simulink model "Model_6DOF_B3"  (R2020b)
settings: Solver=FixedStepAuto  StartTime=0.0  StopTime=120  FixedStep=0.05  RelTol=1e-3
values from neighbouring files (symbols this model uses):
  Ba_0 = [0 0 0 0 0 0]    [ctrl_mode_param.m]
  Bb = 4418825.3321    [load_data.m]
  Bv_0 = [tgt_speed 0 0 0 0 0]    [ctrl_mode_param.m]
  Bx_0 = [0 0 tgt_depth 0 0 0]    [ctrl_mode_param.m]
  Ixx = 5.23e7    (= 52300000)    [load_data.m]
  Ixy = 0    [load_data.m]
  Ixz = 0    [load_data.m]
  Iyy = 1.375e9    (= 1375000000)    [load_data.m]
  Iyz = 0    [load_data.m]
  Izz = 1.367e9    (= 1367000000)    [load_data.m]
  Mb = 4418825.3321    [load_data.m]
  Xb = 0    [load_data.m]
  Xg = 0    [load_data.m]
  Yb = 0    [load_data.m]
  Yg = 0    [load_data.m]
  Zb = 0.4406    [load_data.m]
  Zg = 0    [load_data.m]
undefined symbols (not defined in the file or in its folder): dA_BP1, dA_BP2, dA_Hull, dA_PH, dA_Sail, dA_SProot, dA_X1a, dA_X1b, dA_X2a, dA_X2b, dA_X3a, dA_X3b, dA_X4a, dA_X4b, its, n_BP1, n_BP2, n_Hull, n_PH, n_Sail, n_SProot, n_X1a, n_X1b, n_X2a, n_X2b, n_X3a, n_X3b, n_X4a, n_X4b, nt_BP1, nt_BP2, nt_Hull, nt_PH, nt_Sail, nt_SProot, nt_X1a, nt_X1b, nt_X2a, nt_X2b, nt_X3a, nt_X3b, nt_X4a, nt_X4b, Usp, vt1_BP1, vt1_BP2, vt1_Hull, vt1_PH, vt1_Sail, vt1_SProot, vt1_X1a, vt1_X1b, vt1_X2a, vt1_X2b, vt1_X3a, vt1_X3b, vt1_X4a, vt1_X4b, vt2_BP1, vt2_BP2 ... (+27)
libraries: simulink x5
(part 4 of 15)

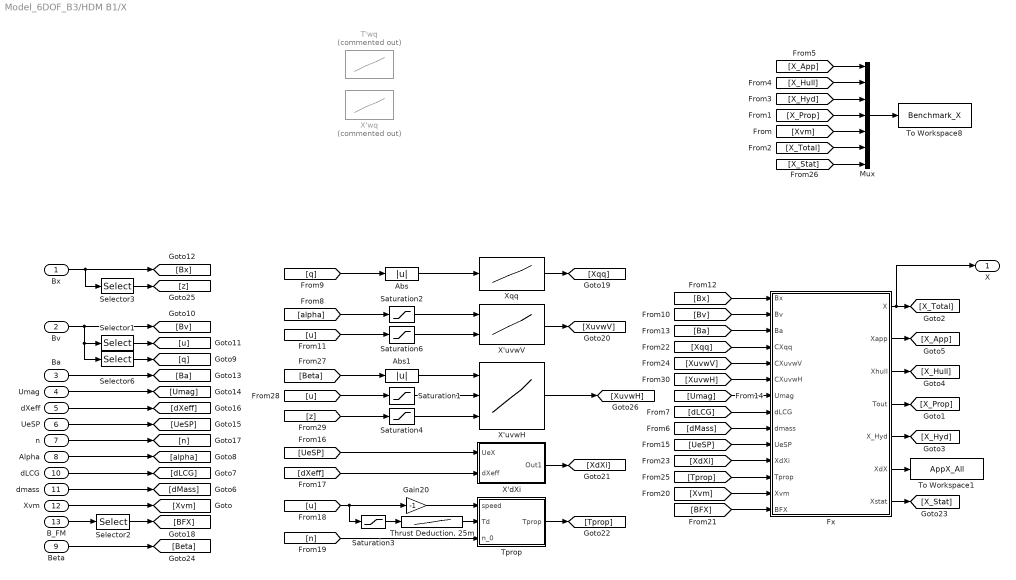
== system Model_6DOF_B3/HDM B1/X ==
  Bx : Inport
  Bv : Inport  Port=2
  Ba : Inport  Port=3
  Umag : Inport  Port=4
  dXeff : Inport  Port=5
  UeSP : Inport  Port=6
  n : Inport  Port=7
  Alpha : Inport  Port=8
  Beta : Inport  Port=9
  dLCG : Inport  Port=10
  dmass : Inport  Port=11
  Xvm : Inport  Port=12
  B_FM : Inport  Port=13
  Abs : Abs
  Abs1 : Abs
  Fx : MATLAB Function  TreatAsAtomicUnit=on
  Gain20 : Gain  Gain=-1
  Mux : Mux  Inputs=7
  Saturation1 : Saturate  UpperLimit=-1.543332  LowerLimit=-5.14444
  Saturation2 : Saturate  UpperLimit=30  LowerLimit=-30
  Saturation3 : Saturate  UpperLimit=-1.54333333  LowerLimit=-5.1444
  Saturation4 : Saturate  UpperLimit=-13.8724  LowerLimit=-35.0624
  Saturation6 : Saturate  UpperLimit=-1.543332  LowerLimit=-5.14444
  Selector1 : Selector  InputPortWidth=6  IndexOptions=Index vector (dialog)  Indices=1  OutputSizes=1
  Selector2 : Selector  InputPortWidth=6  IndexOptions=Index vector (dialog)  Indices=1  OutputSizes=1
  Selector3 : Selector  InputPortWidth=6  IndexOptions=Index vector (dialog)  Indices=3  OutputSizes=1
  Selector6 : Selector  InputPortWidth=6  IndexOptions=Index vector (dialog)  Indices=5  OutputSizes=1
  T'wq : Lookup_n-D  Commented=on  BreakpointsForDimension1=|  BreakpointsForDimension2=|  Table=|  InternalRulePriority=Speed  RndMeth=Simplest  InputSameDT=on
      BreakpointsForDimension1=|
      | [-2.5000E-02
      | -2.0000E-02
      | -1.5000E-02
      | -1.0000E-02
      | -5.0000E-03
      | 0.0000E+00
      | 5.0000E-03
      | ]
      BreakpointsForDimension2=|
      | [-7.71666
      | -5.14444
      | -3.086664]
      Table=|
      | reshape([-2.7354E-04
      | -2.2597E-04
      | -1.7840E-04
      | -1.3083E-04
      | -8.3252E-05
      | -3.5680E-05
      | 1.1893E-05
      | -9.4081E-05
      | -7.5784E-05
      | -5.7487E-05
      | -3.9189E-05
      | -2.0892E-05
      | -2.5949E-06
      | 1.5702E-05
      | -1.4962E-04
      | -1.2035E-04
      | -9.1070E-05
      | -6.1795E-05
      | -3.2519E-05
      | -3.2436E-06
      | 2.6032E-05
      | ],[7,3])
      settings: InputPortMap=u0,u1
  "Thrust Deduction, 25m" : Lookup_n-D  NumberOfTableDimensions=1  BreakpointsForDimension1=[-5.14444,-3.086664,-1.543332]  BreakpointsForDimension2=[0.1 1.543332 3.086664 5.14444 100]  Table=[0.2496,0.2444134,0.245958]  InternalRulePriority=Speed  RndMeth=Simplest  InputSameDT=on
  To Workspace1 : ToWorkspace  VariableName=AppX_All  SaveFormat=Timeseries  SampleTime=-1
  To Workspace8 : ToWorkspace  VariableName=Benchmark_X  SaveFormat=Timeseries  SampleTime=-1
  Tprop : MATLAB Function  TreatAsAtomicUnit=on
  X'dXi : Subsystem
  X'uvwH : Lookup_n-D  NumberOfTableDimensions=3  BreakpointsForDimension1=|  BreakpointsForDimension2=|  BreakpointsForDimension3=|  Table=|  InternalRulePriority=Speed  RndMeth=Simplest  InputSameDT=on
      BreakpointsForDimension1=|
      | [0
      | 4
      | 8
      | 12]
      BreakpointsForDimension2=|
      | [-5.1444
      | -3.08664
      | -1.54332]
      Table=|
      | reshape([0.0000000E+00
      | 8.7490400E-05
      | -4.2970032E-04
      | -8.6882993E-04
      | 0.0000000E+00
      | 9.2255510E-05
      | -3.6462757E-04
      | -8.6516720E-04
      | 0.0000000E+00
      | -8.0508235E-05
      | -3.3610820E-04
      | -9.1603355E-04
      | 0.0000000E+00
      | -9.0915847E-05
      | -3.9252667E-04
      | -9.2068441E-04
      | 0.0000000E+00
      | -1.0407599E-04
      | -3.8836462E-04
      | -9.1865822E-04
      | 0.0000000E+00
      | -8.4723950E-05
      | -3.5324770E-04
      | -9.7126434E-04
      | 0.0000000E+00
      | -9.3766627E-05
      | -4.1342843E-04
      | -9.4161914E-04
      | 0.0000000E+00
      | -1.0916277E-04
      | -4.0683220E-04
      | -9.6707684E-04
      | 0.0000000E+00
      | -8.8664811E-05
      | -3.7605406E-04
      | -9.4194453E-04
      | 0.0000000E+00
      | -9.2876985E-05
      | -4.0365964E-04
      | -9.3239814E-04
      | 0.0000000E+00
      | -1.1414747E-04
      | -4.4323139E-04
      | -1.0049645E-03
      | 0.0000000E+00
      | -9.4615234E-05
      | -4.9251136E-04
      | -9.8471513E-04],[4,3,4])
      BreakpointsForDimension3=|
      | [-35.0624 -18.3724 -15.3724 -13.8724
      | ]
      settings: InputPortMap=u0,u1,u2
  X'uvwV : Lookup_n-D  BreakpointsForDimension1=|  BreakpointsForDimension2=|  Table=|  InternalRulePriority=Speed  RndMeth=Simplest  InputSameDT=on
      BreakpointsForDimension1=|
      | [-12
      | -8
      | -4
      | 0
      | 4
      | 8
      | 12]
      BreakpointsForDimension2=|
      | [-5.1444
      | -3.08664
      | -1.54332]
      Table=|
      | reshape([8.5556500E-04
      | 9.0045500E-04
      | 9.7379500E-04
      | 1.0292250E-03
      | 1.0286950E-03
      | 9.7963500E-04
      | 1.0147450E-03
      | 9.0637500E-04
      | 9.3710500E-04
      | 1.0133950E-03
      | 1.0723650E-03
      | 1.0693650E-03
      | 1.0284650E-03
      | 1.1084650E-03
      | 9.8653120E-04
      | 9.9350120E-04
      | 1.0534412E-03
      | 1.1098412E-03
      | 1.1115412E-03
      | 1.0836412E-03
      | 1.1582412E-03],[7,3])
      settings: InputPortMap=u0,u1
  X'wq : Lookup_n-D  Commented=on  BreakpointsForDimension1=|  BreakpointsForDimension2=[-7.71666 -5.14444 -3.086664 -1.543332]  Table=|  InternalRulePriority=Speed  RndMeth=Simplest  InputSameDT=on
      BreakpointsForDimension1=|
      | [-2.5000E-02
      | -2.0000E-02
      | -1.5000E-02
      | -1.0000E-02
      | -5.0000E-03
      | 0.0000E+00
      | 5.0000E-03
      | ]
      Table=|
      | reshape([2.0716E-04
      | 1.9060E-04
      | 1.7404E-04
      | 1.5748E-04
      | 1.4091E-04
      | 1.2435E-04
      | 1.0779E-04
      | 1.3610E-04
      | 1.1954E-04
      | 1.0298E-04
      | 8.6416E-05
      | 6.9855E-05
      | 5.3295E-05
      | 3.6734E-05
      | 1.5577E-04
      | 1.2817E-04
      | 1.0057E-04
      | 7.2967E-05
      | 4.5366E-05
      | 1.7765E-05
      | -9.8361E-06
      | 1.4245E-04
      | 1.1485E-04
      | 8.7244E-05
      | 5.9643E-05
      | 3.2042E-05
      | 4.4412E-06
      | -2.3160E-05
      | ],[7,4])
      settings: InputPortMap=u0,u1
  Xqq : Lookup_n-D  NumberOfTableDimensions=1  BreakpointsForDimension1=|  Table=|  InternalRulePriority=Speed  RndMeth=Simplest  InputSameDT=on
      BreakpointsForDimension1=|
      | [-0.02
      | -0.015
      | -0.012958963
      | -0.009719222
      | -0.006479482
      | -0.003239741
      | -0.00161987
      | -0.000647948
      | 0.000647948
      | 0.00161987
      | 0.003239741
      | 0.006479482
      | 0.009719222
      | 0.012958963
      | 0.015
      | 0.02
      | ]
      Table=|
      | [1.5581E-04
      | 1.1369E-04
      | 2.0348E-04
      | 4.5268E-04
      | 3.8456E-04
      | 9.9241E-05
      | 3.8998E-04
      | 9.1300E-05
      | -3.1574E-04
      | -7.9139E-05
      | -9.0517E-04
      | -4.4764E-04
      | -5.9612E-04
      | -5.5873E-04
      | -5.9343E-04
      | -5.5869E-04
      | ]
  X : Outport
  wires:
  [XuvwH] -> Fx/6(CXuvwH)
  X'uvwH/1 -> [XuvwH]
  Saturation4/1 -> X'uvwH/3
  [z] -> Saturation4/1
  Selector3/1 -> [z]
  Saturation1/1 -> X'uvwH/2
  [u] -> Saturation1/1
  [Beta] -> Abs1/1
  Abs1/1 -> X'uvwH/1
  Beta/1 -> [Beta]
  [X_Stat] -> Mux/7
  [Tprop] -> Fx/12(Tprop)
  Tprop/1(Tprop) -> [Tprop]
  [XuvwV] -> Fx/5(CXuvwV)
  [XdXi] -> Fx/11(XdXi)
  X'dXi/1(Out1) -> [XdXi]
  X'uvwV/1 -> [XuvwV]
  Xqq/1 -> [Xqq]
  [Xqq] -> Fx/4(CXqq)
  [BFX] -> Fx/14(BFX)
  Selector2/1 -> [BFX]
  [Xvm] -> Fx/13(Xvm)
  Xvm/1 -> [Xvm]
  [n] -> Tprop/3(n_0)
  n/1 -> [n]
  dXeff/1 -> [dXeff]
  [dXeff] -> X'dXi/2(dXeff)
  [UeSP] -> X'dXi/1(UeX)
  UeSP/1 -> [UeSP]
  [UeSP] -> Fx/10(UeSP)
  Umag/1 -> [Umag]
  [Umag] -> Fx/7(Umag)
  Ba/1 -> [Ba]
  [Ba] -> Fx/3(Ba)
  Bx/1 -> Selector3/1, [Bx]
  [Bx] -> Fx/1(Bx)
  Selector1/1 -> [u]
  [u] -> Saturation6/1
  [Bv] -> Fx/2(Bv)
  Selector6/1 -> [q]
  Bv/1 -> Selector1/1, Selector6/1, [Bv]
  Alpha/1 -> [alpha]
  [alpha] -> Saturation2/1
  dLCG/1 -> [dLCG]
  [dLCG] -> Fx/8(dLCG)
  dmass/1 -> [dMass]
  [dMass] -> Fx/9(dmass)
  [X_App] -> Mux/1
  Fx/2(Xapp) -> [X_App]
  Fx/3(Xhull) -> [X_Hull]
  [X_Hull] -> Mux/2
  Fx/5(X_Hyd) -> [X_Hyd]
  [X_Hyd] -> Mux/3
  [X_Total] -> Mux/6
  [X_Prop] -> Mux/4
  Fx/4(Tout) -> [X_Prop]
  [Xvm] -> Mux/5
  Fx/7(Xstat) -> [X_Stat]
  B_FM/1 -> Selector2/1
  Fx/6(XdX) -> To Workspace1/1
  Mux/1 -> To Workspace8/1
  Saturation6/1 -> X'uvwV/2
  "Thrust Deduction, 25m"/1 -> Tprop/2(Td)
  Saturation3/1 -> "Thrust Deduction, 25m"/1
  Abs/1 -> Xqq/1
  [q] -> Abs/1
  [u] -> Gain20/1, Saturation3/1
  Fx/1(X) -> X/1, [X_Total]
  Gain20/1 -> Tprop/1(speed)
  Saturation2/1 -> X'uvwV/1

== system Model_6DOF_B3/HDM B1/X 6d org ==
  Bx : Inport
  Bv : Inport  Port=2
  Ba : Inport  Port=3
  Umag : Inport  Port=4
  dXeff : Inport  Port=5
  UeX : Inport  Port=6
  n : Inport  Port=7
  Alpha : Inport  Port=8
  dLCG : Inport  Port=9
  dmass : Inport  Port=10
  Xvm : Inport  Port=11
  Fx : MATLAB Function  TreatAsAtomicUnit=on
  Gain20 : Gain  Gain=-1
  MATLAB Function2 : MATLAB Function  TreatAsAtomicUnit=on
  Product3 : Product
  Saturation1 : Saturate  UpperLimit=-1  LowerLimit=-7.782
  Saturation2 : Saturate  UpperLimit=30  LowerLimit=-30
  Saturation3 : Saturate  UpperLimit=-1.54333333  LowerLimit=-7.782
  Selector : Selector  InputPortWidth=6  IndexOptions=Index vector (dialog)  Indices=1  OutputSizes=1
  Selector1 : Selector  InputPortWidth=6  IndexOptions=Index vector (dialog)  Indices=3  OutputSizes=1
  Selector18 : Selector  InputPortWidth=6  IndexOptions=Index vector (dialog)  Indices=1  OutputSizes=1
  Selector19 : Selector  InputPortWidth=6  IndexOptions=Index vector (dialog)  Indices=1  OutputSizes=1
  Selector2 : Selector  InputPortWidth=6  IndexOptions=Index vector (dialog)  Indices=3  OutputSizes=1
  Selector6 : Selector  InputPortWidth=6  IndexOptions=Index vector (dialog)  Indices=5  OutputSizes=1
  Subsystem1 : Subsystem
  T'wq : Lookup_n-D  BreakpointsForDimension1=|  BreakpointsForDimension2=|  Table=|  InternalRulePriority=Speed  RndMeth=Simplest  InputSameDT=on
      BreakpointsForDimension1=|
      | [-2.5000E-02
      | -2.0000E-02
      | -1.5000E-02
      | -1.0000E-02
      | -5.0000E-03
      | 0.0000E+00
      | 5.0000E-03
      | ]
      BreakpointsForDimension2=|
      | [-7.71666
      | -5.14444
      | -3.086664]
      Table=|
      | reshape([-2.7354E-04
      | -2.2597E-04
      | -1.7840E-04
      | -1.3083E-04
      | -8.3252E-05
      | -3.5680E-05
      | 1.1893E-05
      | -9.4081E-05
      | -7.5784E-05
      | -5.7487E-05
      | -3.9189E-05
      | -2.0892E-05
      | -2.5949E-06
      | 1.5702E-05
      | -1.4962E-04
      | -1.2035E-04
      | -9.1070E-05
      | -6.1795E-05
      | -3.2519E-05
      | -3.2436E-06
      | 2.6032E-05
      | ],[7,3])
      settings: InputPortMap=u0,u1
  "Thrust Deduction, 25m" : Lookup_n-D  NumberOfTableDimensions=1  BreakpointsForDimension1=[-5.14444,-3.086664,-1.543332]  BreakpointsForDimension2=[0.1 1.543332 3.086664 5.14444 100]  Table=[0.2496,0.2444134,0.245958]  InternalRulePriority=Speed  RndMeth=Simplest  InputSameDT=on
  To Workspace : ToWorkspace  VariableName=Xapp  SaveFormat=Timeseries  SampleTime=-1
  To Workspace1 : ToWorkspace  VariableName=Xstat  SaveFormat=Timeseries  SampleTime=-1
  To Workspace2 : ToWorkspace  VariableName=Xhull  SaveFormat=Timeseries  SampleTime=-1
  To Workspace3 : ToWorkspace  VariableName=Tout  SaveFormat=Timeseries  SampleTime=-1
  To Workspace4 : ToWorkspace  VariableName=Xtotal  SaveFormat=Timeseries  SampleTime=-1
  Tprop : MATLAB Function  TreatAsAtomicUnit=on
  X'uvw : Lookup_n-D  BreakpointsForDimension1=|  BreakpointsForDimension2=|  Table=|  InternalRulePriority=Speed  RndMeth=Simplest  InputSameDT=on
      BreakpointsForDimension1=|
      | [-12
      | -8
      | -4
      | 0
      | 4
      | 8
      | 12]
      BreakpointsForDimension2=|
      | [-5.1444
      | -3.08664
      | -1.54332]
      Table=|
      | reshape([8.0227E-04
      | 8.4716E-04
      | 9.2050E-04
      | 9.7593E-04
      | 9.7540E-04
      | 9.2634E-04
      | 9.6145E-04
      | 8.8861E-04
      | 9.1934E-04
      | 9.9563E-04
      | 1.0546E-03
      | 1.0516E-03
      | 1.0107E-03
      | 1.0907E-03
      | 9.8209E-04
      | 9.8906E-04
      | 1.0490E-03
      | 1.1054E-03
      | 1.1071E-03
      | 1.0792E-03
      | 1.1538E-03],[7,3])
      settings: InputPortMap=u0,u1
  X'wq : Lookup_n-D  BreakpointsForDimension1=|  BreakpointsForDimension2=[-7.71666 -5.14444 -3.086664 -1.543332]  Table=|  InternalRulePriority=Speed  RndMeth=Simplest  InputSameDT=on
      BreakpointsForDimension1=|
      | [-2.5000E-02
      | -2.0000E-02
      | -1.5000E-02
      | -1.0000E-02
      | -5.0000E-03
      | 0.0000E+00
      | 5.0000E-03
      | ]
      Table=|
      | reshape([2.0716E-04
      | 1.9060E-04
      | 1.7404E-04
      | 1.5748E-04
      | 1.4091E-04
      | 1.2435E-04
      | 1.0779E-04
      | 1.3610E-04
      | 1.1954E-04
      | 1.0298E-04
      | 8.6416E-05
      | 6.9855E-05
      | 5.3295E-05
      | 3.6734E-05
      | 1.5577E-04
      | 1.2817E-04
      | 1.0057E-04
      | 7.2967E-05
      | 4.5366E-05
      | 1.7765E-05
      | -9.8361E-06
      | 1.4245E-04
      | 1.1485E-04
      | 8.7244E-05
      | 5.9643E-05
      | 3.2042E-05
      | 4.4412E-06
      | -2.3160E-05
      | ],[7,4])
      settings: InputPortMap=u0,u1
  Xqq : Lookup_n-D  NumberOfTableDimensions=1  BreakpointsForDimension1=|  Table=|  InternalRulePriority=Speed  RndMeth=Simplest  InputSameDT=on
      BreakpointsForDimension1=|
      | [-0.02
      | -0.015
      | -0.012958963
      | -0.009719222
      | -0.006479482
      | -0.003239741
      | -0.00161987
      | -0.000647948
      | 0.000647948
      | 0.00161987
      | 0.003239741
      | 0.006479482
      | 0.009719222
      | 0.012958963
      | 0.015
      | 0.02
      | ]
      Table=|
      | [1.5581E-04
      | 1.1369E-04
      | 2.0348E-04
      | 4.5268E-04
      | 3.8456E-04
      | 9.9241E-05
      | 3.8998E-04
      | 9.1300E-05
      | -3.1574E-04
      | -7.9139E-05
      | -9.0517E-04
      | -4.4764E-04
      | -5.9612E-04
      | -5.5873E-04
      | -5.9343E-04
      | -5.5869E-04
      | ]
  X : Outport
  wires:
  Selector2/1 -> Subsystem1/3(z)
  Fx/5(Tout) -> To Workspace3/1
  Fx/4(Xhull) -> To Workspace2/1
  Fx/3(Xstat) -> To Workspace1/1
  Fx/2(Xapp) -> To Workspace/1
  Xvm/1 -> Fx/14(Xvm)
  X'uvw/1 -> Fx/6(CXuvw)
  T'wq/1 -> Fx/7(CTwq)
  X'wq/1 -> Fx/5(CXwq)
  dXeff/1 -> Subsystem1/2(dXeff)
  Selector1/1 -> Product3/2
  Product3/1 -> T'wq/1, X'wq/1
  Saturation1/1 -> T'wq/2, X'uvw/2, X'wq/2
  Subsystem1/1(XdXi) -> Fx/12(XdXi)
  dmass/1 -> Fx/10(dmass)
  dLCG/1 -> Fx/9(dLCG)
  n/1 -> Tprop/3(n_0)
  Ba/1 -> Fx/3(Ba)
  Bx/1 -> Selector2/1, Fx/1(Bx)
  Saturation2/1 -> X'uvw/1
  Selector18/1 -> Saturation1/1
  Selector/1 -> Gain20/1
  Gain20/1 -> Tprop/1(speed)
  Fx/1(X) -> X/1, To Workspace4/1
  Selector19/1 -> Saturation3/1
  Selector6/1 -> Product3/1, MATLAB Function2/1(u)
  Umag/1 -> Fx/8(Umag)
  MATLAB Function2/1(y) -> Xqq/1
  Alpha/1 -> Saturation2/1
  Bv/1 -> Fx/2(Bv), Selector6/1, Selector1/1, Selector18/1, Selector/1, Selector19/1
  Xqq/1 -> Fx/4(CXqq)
  Saturation3/1 -> "Thrust Deduction, 25m"/1
  "Thrust Deduction, 25m"/1 -> Tprop/2(Td)
  UeX/1 -> Fx/11(UeX), Subsystem1/1(UeX)
  Tprop/1(Tprop) -> Fx/13(Tprop)

== system Model_6DOF_B3/HDM B1/Y ==
  Bx : Inport
  Bv : Inport  Port=2
  Ba : Inport  Port=3
  Beta : Inport  Port=4
  Umag : Inport  Port=5
  dX : Inport  Port=6
  UeX : Inport  Port=7
  dLCG : Inport  Port=8
  dmass : Inport  Port=9
  Yvm : Inport  Port=10
  BFM : Inport  Port=11
  Abs1 : Abs
  Abs2 : Abs
  Fy : MATLAB Function  TreatAsAtomicUnit=on
  Gain1 : Gain
  Gain2 : Gain  Gain=2
  Mux : Mux  Inputs=7
  Product{,1..3} (4 alike) : Product
  Saturation4 : Saturate  UpperLimit=-13.8724  LowerLimit=-35.0624
  Selector1 : Selector  InputPortWidth=6  IndexOptions=Index vector (dialog)  Indices=2  OutputSizes=1
  Selector2 : Selector  InputPortWidth=6  IndexOptions=Index vector (dialog)  Indices=6  OutputSizes=1
  Selector3 : Selector  InputPortWidth=6  IndexOptions=Index vector (dialog)  Indices=2  OutputSizes=1
  Selector4 : Selector  InputPortWidth=6  IndexOptions=Index vector (dialog)  Indices=3  OutputSizes=1
  Selector7 : Selector  InputPortWidth=6  IndexOptions=Index vector (dialog)  Indices=1  OutputSizes=1
  Sign : Signum
  Sign1 : Signum
  To Workspace1 : ToWorkspace  VariableName=AppY_All  SaveFormat=Timeseries  SampleTime=-1
  To Workspace2 : ToWorkspace  VariableName=FYHullVM  SaveFormat=Timeseries  SampleTime=-1
  To Workspace8 : ToWorkspace  VariableName=Benchmark_Y  SaveFormat=Timeseries  SampleTime=-1
  Y'ur : Lookup_n-D  NumberOfTableDimensions=1  BreakpointsForDimension1=|  Table=|  InternalRulePriority=Speed  RndMeth=Simplest  InputSameDT=on
      BreakpointsForDimension1=|
      | [0.03999989
      | 0.079999993
      | 0.11999963
      | 0.15999956]
      Table=|
      | [-5.2094E-04
      | -1.0594E-03
      | -1.5649E-03
      | -2.0981E-03]
  Y'uvw : Lookup_n-D  NumberOfTableDimensions=3  BreakpointsForDimension1=|  BreakpointsForDimension2=|  BreakpointsForDimension3=|  Table=|  InternalRulePriority=Speed  RndMeth=Simplest  InputSameDT=on
      BreakpointsForDimension1=|
      | [0
      | 4
      | 8
      | 12]
      BreakpointsForDimension2=|
      | [-5.1444E+00
      | -3.0866E+00
      | -1.5433E+00
      | ]
      Table=|
      | reshape([0.0000000E+00
      | -5.0280621E-03
      | -9.4175348E-03
      | -1.4397458E-02
      | 0.0000000E+00
      | -5.0037454E-03
      | -9.1645405E-03
      | -1.4507402E-02
      | 0.0000000E+00
      | -4.2819107E-03
      | -9.0361786E-03
      | -1.4507235E-02
      | 0.0000000E+00
      | -4.7723270E-03
      | -9.7378407E-03
      | -1.5377541E-02
      | 0.0000000E+00
      | -4.7276301E-03
      | -9.6949815E-03
      | -1.5393721E-02
      | 0.0000000E+00
      | -4.5359209E-03
      | -9.4966039E-03
      | -1.6947859E-02
      | 0.0000000E+00
      | -5.1295007E-03
      | -1.0575377E-02
      | -1.6672924E-02
      | 0.0000000E+00
      | -4.9811404E-03
      | -1.0209461E-02
      | -1.6298327E-02
      | 0.0000000E+00
      | -4.7780219E-03
      | -1.0008968E-02
      | -1.6115181E-02
      | 0.0000000E+00
      | -5.7252015E-03
      | -1.1973447E-02
      | -1.9152812E-02
      | 0.0000000E+00
      | -5.2128737E-03
      | -1.0845978E-02
      | -1.7281669E-02
      | 0.0000000E+00
      | -4.9979037E-03
      | -1.0845685E-02
      | -1.6944141E-02],[4,3,4])
      BreakpointsForDimension3=|
      | [-35.0624 -18.3724 -15.3724 -13.8724
      | ]
      settings: InputPortMap=u0,u1,u2
  Y'|v|r : Lookup_n-D  NumberOfTableDimensions=1  BreakpointsForDimension1=|  Table=|  InternalRulePriority=Speed  RndMeth=Simplest  InputSameDT=on
      BreakpointsForDimension1=|
      | [-0.0015
      | -0.0012
      | -0.0009
      | -0.0006
      | -0.0003
      | -0.0001
      | 0.0001
      | 0.0003
      | 0.0006
      | 0.0009
      | 0.0012
      | 0.0015]
      Table=|
      | [-2.9784E-01
      | -2.6725E-01
      | -2.3292E-01
      | -2.0077E-01
      | -1.1489E-01
      | -7.6673E-03
      | -7.5516E-03
      | -1.1617E-01
      | -2.0077E-01
      | -2.9128E-01
      | -3.5974E-01
      | -4.7839E-01]
  YdXi : Subsystem
  Y|r|r : Lookup_n-D  NumberOfTableDimensions=1  BreakpointsForDimension1=|  Table=|  InternalRulePriority=Speed  RndMeth=Simplest  InputSameDT=on
      BreakpointsForDimension1=|
      | [-0.02
      | -0.015
      | -0.012958963
      | -0.009719222
      | -0.006479482
      | -0.003239741
      | -0.00161987
      | -0.000647948
      | 0.000647948
      | 0.00161987
      | 0.003239741
      | 0.006479482
      | 0.009719222
      | 0.012958963
      | 0.015
      | 0.02
      | ]
      Table=|
      | [3.6478E-03
      | 3.8686E-03
      | 3.4313E-03
      | 4.0790E-03
      | 3.9500E-03
      | 3.6018E-03
      | 3.6796E-03
      | 3.5502E-03
      | 3.4310E-03
      | 3.4872E-03
      | 4.2239E-03
      | 4.0934E-03
      | 3.0314E-03
      | 2.5726E-03
      | 2.9188E-03
      | 2.7740E-03
      | ]
  Y : Outport
  wires:
  Gain1/1 -> Fy/12(CYdXi)
  Saturation4/1 -> YdXi/2(z), Y'uvw/3  "z"
  Fy/7(FYHullVM) -> To Workspace2/1
  Selector1/1 -> Fy/14(BFY), Mux/7
  BFM/1 -> Selector1/1
  Fy/6(FYAppAll) -> To Workspace1/1
  Fy/5(FYprop) -> Mux/4
  Fy/4(FY_hyd) -> Mux/3
  Fy/3(FYhull) -> Mux/2
  Fy/2(FYApp) -> Mux/1
  Mux/1 -> To Workspace8/1
  Yvm/1 -> Fy/13(Yvm), Mux/5
  Gain2/1 -> Fy/7(CYuvw)
  Product/1 -> Gain2/1
  YdXi/1(YdX) -> Gain1/1
  Abs2/1 -> Y'ur/1
  Sign1/1 -> Product2/1
  Product2/1 -> Fy/5(CYvr)
  Abs1/1 -> Y'uvw/1
  Sign/1 -> Product/1
  Y'uvw/1 -> Product/2
  Selector4/1 -> Saturation4/1
  Y'ur/1 -> Product2/2
  Y|r|r/1 -> Fy/4(CYr)
  Fy/1(Fy) -> Y/1, Mux/6
  Y'|v|r/1 -> Fy/6(CYrr)
  Selector2/1 -> Y|r|r/1, Product3/1, Product1/1
  Product1/1 -> Y'|v|r/1
  Product3/1 -> Sign1/1, Abs2/1
  dX/1 -> YdXi/1(dX)
  dmass/1 -> Fy/11(dmass)
  dLCG/1 -> Fy/10(dLCG)
  Ba/1 -> Fy/3(Ba)
  Selector3/1 -> Product1/2
  UeX/1 -> Fy/9(UeX)
  Bx/1 -> Fy/1(Bx), Selector4/1
  Umag/1 -> Fy/8(Umag)
  Bv/1 -> Fy/2(Bv), Selector2/1, Selector3/1, Selector7/1
  Beta/1 -> Abs1/1, Sign/1
  Selector7/1 -> Y'uvw/2, Product3/2

== system Model_6DOF_B3/HDM B1/Z ==
  Bx : Inport
  Bv : Inport  Port=2
  Ba : Inport  Port=3
  Alpha : Inport  Port=4
  Umag : Inport  Port=5
  dX : Inport  Port=6
  UeSP : Inport  Port=7
  dLCG : Inport  Port=8
  dmass : Inport  Port=9
  Zvm : Inport  Port=10
  BFM : Inport  Port=11
  Fz : MATLAB Function  TreatAsAtomicUnit=on
  Gain : Gain
  Gain2 : Gain
  Linearized Zuvw : MATLAB Function  Commented=on  TreatAsAtomicUnit=on
  Mux1 : Mux  Inputs=6
  Product1 : Product
  Product3 : Product
  Saturation1 : Saturate  UpperLimit=0.04  LowerLimit=-0.04
  Saturation2 : Saturate  UpperLimit=0.0015  LowerLimit=-0.0015
  Saturation3 : Saturate  UpperLimit=0.02  LowerLimit=-0.02
  Saturation4 : Saturate  UpperLimit=-13.8724  LowerLimit=-35.0624
  Saturation5 : Saturate  UpperLimit=-1.5433E+00  LowerLimit=-5.14444
  Selector1 : Selector  InputPortWidth=6  IndexOptions=Index vector (dialog)  Indices=3  OutputSizes=1
  Selector2 : Selector  InputPortWidth=6  IndexOptions=Index vector (dialog)  Indices=5  OutputSizes=1
  Selector3 : Selector  InputPortWidth=6  IndexOptions=Index vector (dialog)  Indices=3  OutputSizes=1
  Selector4 : Selector  InputPortWidth=6  IndexOptions=Index vector (dialog)  Indices=3  OutputSizes=1
  Selector7 : Selector  InputPortWidth=6  IndexOptions=Index vector (dialog)  Indices=1  OutputSizes=1
  To Workspace1 : ToWorkspace  Commented=on  VariableName=Z_stat  SaveFormat=Timeseries  SampleTime=-1
  To Workspace2 : ToWorkspace  VariableName=Benchmark_Z  SaveFormat=Timeseries  SampleTime=-1
  To Workspace3 : ToWorkspace  VariableName=AppZ_All  SaveFormat=Timeseries  SampleTime=-1
  Z'dX : Scope
  Z'uq Prop : Lookup_n-D  BreakpointsForDimension1=|  BreakpointsForDimension2=[-7.71666 -5.14444 -3.086664 -1.543332]  Table=|  InternalRulePriority=Speed  RndMeth=Simplest  InputSameDT=on
      BreakpointsForDimension1=|
      | [-2.0E-01
      | -1.5E-01
      | -1.0E-01
      | -5.0E-02
      | 0.0E+00
      | 5.0E-02
      | 1.0E-01
      | 1.5E-01
      | 2.0E-01
      | ]
      Table=|
      | reshape([1.3913E-04
      | 1.0452E-04
      | 6.9900E-05
      | 3.5283E-05
      | 6.6700E-07
      | -3.3949E-05
      | -6.8566E-05
      | -1.0318E-04
      | -1.3780E-04
      | 2.8914E-04
      | 2.1702E-04
      | 1.4490E-04
      | 7.2785E-05
      | 6.6700E-07
      | -7.1451E-05
      | -1.4357E-04
      | -2.1569E-04
      | -2.8780E-04
      | 1.1606E-04
      | 8.7208E-05
      | 5.8361E-05
      | 2.9514E-05
      | 6.6700E-07
      | -2.8180E-05
      | -5.7027E-05
      | -8.5874E-05
      | -1.1472E-04
      | 1.1606E-04
      | 8.7208E-05
      | 5.8361E-05
      | 2.9514E-05
      | 6.6700E-07
      | -2.8180E-05
      | -5.7027E-05
      | -8.5874E-05
      | -1.1472E-04],[9,4])
      settings: InputPortMap=u0,u1
  Z'uvw : Lookup_n-D  NumberOfTableDimensions=3  BreakpointsForDimension1=|  BreakpointsForDimension2=|  BreakpointsForDimension3=|  Table=|  InternalRulePriority=Speed  RndMeth=Simplest  InputSameDT=on
      BreakpointsForDimension1=|
      | [-12
      | -8
      | -4
      | 0
      | 4
      | 8
      | 12]
      BreakpointsForDimension2=|
      | [-5.1444E+00
      | -3.0866E+00
      | -1.5433E+00
      | ]
      Table=|
      | reshape([-3.82587E-03
      | -2.42543E-03
      | -1.05453E-03
      | 1.94202E-04
      | 1.48991E-03
      | 3.04047E-03
      | 4.14104E-03
      | -3.76348E-03
      | -2.38508E-03
      | -9.82619E-04
      | 1.94202E-04
      | 1.47560E-03
      | 3.02863E-03
      | 4.06663E-03
      | -3.75964E-03
      | -2.29001E-03
      | -8.34074E-04
      | 1.94202E-04
      | 1.38956E-03
      | 2.91153E-03
      | 4.15251E-03
      | -3.11218E-03
      | -1.80502E-03
      | -4.97855E-04
      | 8.09305E-04
      | 2.11647E-03
      | 3.42363E-03
      | 4.73079E-03
      | -2.62573E-03
      | -1.48072E-03
      | -3.35708E-04
      | 8.09305E-04
      | 1.95432E-03
      | 3.09933E-03
      | 4.24434E-03
      | -2.06413E-03
      | -1.10632E-03
      | -1.48507E-04
      | 8.09305E-04
      | 1.76712E-03
      | 2.72493E-03
      | 3.68274E-03
      | -3.09997E-03
      | -1.76300E-03
      | -4.26025E-04
      | 9.10947E-04
      | 2.24792E-03
      | 3.58489E-03
      | 4.92186E-03
      | -2.49055E-03
      | -1.35672E-03
      | -2.22886E-04
      | 9.10947E-04
      | 2.04478E-03
      | 3.17861E-03
      | 4.31245E-03
      | -2.64104E-03
      | -1.45704E-03
      | -2.73048E-04
      | 9.10947E-04
      | 2.09494E-03
      | 3.27894E-03
      | 4.46293E-03
      | -0.003059752
      | -0.001711935
      | -0.000364117
      | 0.0009837
      | 0.002331518
      | 0.003679335
      | 0.005027153
      | -0.002351082
      | -0.0012256
      | -0.000100118
      | 0.0009837
      | 0.002109182
      | 0.003234664
      | 0.004360146
      | -0.001725739
      | -0.000822593
      | 8.05539E-05
      | 0.0009837
      | 0.001886847
      | 0.002789993
      | 0.00369314],[7,3,4])
      BreakpointsForDimension3=|
      | [-35.0624 -18.3724 -15.3724 -13.8724
      | ]
      settings: InputPortMap=u0,u1,u2
  ZdXi : Subsystem
  Zqq : Lookup_n-D  NumberOfTableDimensions=1  BreakpointsForDimension1=|  Table=|  InternalRulePriority=Speed  RndMeth=Simplest  InputSameDT=on
      BreakpointsForDimension1=|
      | [-0.02
      | -0.015
      | -0.012958963
      | -0.009719222
      | -0.006479482
      | -0.003239741
      | -0.00161987
      | -0.000647948
      | 0.000647948
      | 0.00161987
      | 0.003239741
      | 0.006479482
      | 0.009719222
      | 0.012958963
      | 0.015
      | 0.02
      | ]
      Table=|
      | [3.6478E-03
      | 3.8686E-03
      | 3.4313E-03
      | 4.0790E-03
      | 3.9500E-03
      | 3.6018E-03
      | 3.6796E-03
      | 3.5502E-03
      | 3.4310E-03
      | 3.4872E-03
      | 4.2239E-03
      | 4.0934E-03
      | 3.0314E-03
      | 2.5726E-03
      | 2.9188E-03
      | 2.7740E-03
      | ]
  Zuq : Lookup_n-D  NumberOfTableDimensions=1  BreakpointsForDimension1=|  Table=|  InternalRulePriority=Speed  RndMeth=Simplest  InputSameDT=on
      BreakpointsForDimension1=|
      | [-0.04
      | -0.03
      | -0.02
      | -0.01
      | -0.005
      | -0.002
      | 0.002
      | 0.005
      | 0.01
      | 0.02
      | 0.03
      | 0.04
      | ]
      Table=|
      | [-9.8908E-03
      | -9.0784E-03
      | -8.9566E-03
      | -1.0733E-02
      | -1.4141E-02
      | -2.4189E-02
      | -6.5605E-03
      | -7.1594E-03
      | -7.6366E-03
      | -7.9008E-03
      | -6.1794E-03
      | -6.1029E-03
      | ]
  Zwq : Lookup_n-D  NumberOfTableDimensions=1  BreakpointsForDimension1=|  Table=|  InternalRulePriority=Speed  RndMeth=Simplest  InputSameDT=on
      BreakpointsForDimension1=|
      | [-0.0015
      | -0.0012
      | -0.0009
      | -0.0006
      | -0.0003
      | -0.0001
      | 0.0001
      | 0.0003
      | 0.0006
      | 0.0009
      | 0.0012
      | 0.0015]
      Table=|
      | [-2.9784E-01
      | -2.6725E-01
      | -2.3292E-01
      | -2.0077E-01
      | -1.1489E-01
      | -7.6673E-03
      | -7.5516E-03
      | -1.1617E-01
      | -2.0077E-01
      | -2.9128E-01
      | -3.5974E-01
      | -4.7839E-01]
  Z : Outport
  wires:
  Fz/7(FZApp_All) -> To Workspace3/1
  Selector7/1 -> Saturation5/1
  Saturation5/1 -> Z'uq Prop/2, Z'uvw/2, Product3/2
  Saturation4/1 -> Z'uvw/3, ZdXi/2(z)  "dpeth"
  ZdXi/1(ZdX) -> Gain2/1
  Fz/6(FZ_Hyd) -> [Z_Hyd]
  Fz/5(FZProp) -> [Z_Prop]
  Fz/4(FZHull) -> [Z_Hull]
  Fz/2(FZApp) -> [Z_App]
  [Zvm] -> Mux1/5
  [Z_Hyd] -> Mux1/3
  [Z_Total] -> Mux1/6
  [Z_Prop] -> Mux1/4
  Mux1/1 -> To Workspace2/1
  [Z_App] -> Mux1/1
  [Z_Hull] -> Mux1/2
  Gain2/1 -> Fz/13(ZdXi), Z'dX/1
  Selector1/1 -> Fz/15(BFZ)
  BFM/1 -> Selector1/1
  Fz/3(FZStat) -> To Workspace1/1
  Gain/1 -> Fz/7(Zuvw)
  Zqq/1 -> Fz/4(Zqq)
  Z'uq Prop/1 -> Fz/8(CZProp)
  Zwq/1 -> Fz/6(Zwq)
  Selector2/1 -> Product1/1, Saturation3/1, Product3/1
  Alpha/1 -> Z'uvw/1
  Bv/1 -> Fz/2(Bv), Selector7/1, Selector3/1, Selector2/1
  Umag/1 -> Fz/9(Umag)
  Bx/1 -> Fz/1(Bx), Selector4/1
  Product3/1 -> Saturation1/1, Z'uq Prop/1
  UeSP/1 -> Fz/10(UeSP)
  Selector3/1 -> Product1/2
  Product1/1 -> Saturation2/1
  dLCG/1 -> Fz/11(dLCG)
  dmass/1 -> Fz/12(dmass)
  dX/1 -> ZdXi/1(dX)
  Saturation1/1 -> Zuq/1
  Saturation2/1 -> Zwq/1
  Saturation3/1 -> Zqq/1
  Fz/1(Fz) -> [Z_Total], Z/1
  Zuq/1 -> Fz/5(Zuq)
  Ba/1 -> Fz/3(Ba)
  Zvm/1 -> [Zvm], Fz/14(Zvm)
  Selector4/1 -> Saturation4/1
  Z'uvw/1 -> Gain/1

== system Model_6DOF_B3/HDM B1/Z 6d org ==
  Bx : Inport
  Bv : Inport  Port=2
  Ba : Inport  Port=3
  Alpha : Inport  Port=4
  Umag : Inport  Port=5
  dX : Inport  Port=6
  UeX : Inport  Port=7
  dLCG : Inport  Port=8
  dmass : Inport  Port=9
  Zvm : Inport  Port=10
  Fz : MATLAB Function  TreatAsAtomicUnit=on
  Product1 : Product
  Product3 : Product
  Saturation1 : Saturate  UpperLimit=0.04  LowerLimit=-0.04
  Saturation2 : Saturate  UpperLimit=0.0015  LowerLimit=-0.0015
  Saturation3 : Saturate  UpperLimit=0.02  LowerLimit=-0.02
  Selector1 : Selector  InputPortWidth=6  IndexOptions=Index vector (dialog)  Indices=3  OutputSizes=1
  Selector2 : Selector  InputPortWidth=6  IndexOptions=Index vector (dialog)  Indices=5  OutputSizes=1
  Selector3 : Selector  InputPortWidth=6  IndexOptions=Index vector (dialog)  Indices=3  OutputSizes=1
  Selector4 : Selector  InputPortWidth=6  IndexOptions=Index vector (dialog)  Indices=3  OutputSizes=1
  Selector7 : Selector  InputPortWidth=6  IndexOptions=Index vector (dialog)  Indices=1  OutputSizes=1
  To Workspace : ToWorkspace  VariableName=Zapp  SaveFormat=Timeseries  SampleTime=-1
  To Workspace1 : ToWorkspace  VariableName=Ztotal  SaveFormat=Timeseries  SampleTime=-1
  To Workspace2 : ToWorkspace  VariableName=Zstat  SaveFormat=Timeseries  SampleTime=-1
  To Workspace3 : ToWorkspace  VariableName=Zprop  SaveFormat=Timeseries  SampleTime=-1
  To Workspace4 : ToWorkspace  VariableName=Zhull  SaveFormat=Timeseries  SampleTime=-1
  Z'dwdt : MATLAB Function  TreatAsAtomicUnit=on
  Z'uq Prop : Lookup_n-D  BreakpointsForDimension1=|  BreakpointsForDimension2=[-7.71666 -5.14444 -3.086664 -1.543332]  Table=|  InternalRulePriority=Speed  RndMeth=Simplest  InputSameDT=on
      BreakpointsForDimension1=|
      | [-2.0E-01
      | -1.5E-01
      | -1.0E-01
      | -5.0E-02
      | 0.0E+00
      | 5.0E-02
      | 1.0E-01
      | 1.5E-01
      | 2.0E-01
      | ]
      Table=|
      | reshape([1.3913E-04
      | 1.0452E-04
      | 6.9900E-05
      | 3.5283E-05
      | 6.6700E-07
      | -3.3949E-05
      | -6.8566E-05
      | -1.0318E-04
      | -1.3780E-04
      | 2.8914E-04
      | 2.1702E-04
      | 1.4490E-04
      | 7.2785E-05
      | 6.6700E-07
      | -7.1451E-05
      | -1.4357E-04
      | -2.1569E-04
      | -2.8780E-04
      | 1.1606E-04
      | 8.7208E-05
      | 5.8361E-05
      | 2.9514E-05
      | 6.6700E-07
      | -2.8180E-05
      | -5.7027E-05
      | -8.5874E-05
      | -1.1472E-04
      | 1.1606E-04
      | 8.7208E-05
      | 5.8361E-05
      | 2.9514E-05
      | 6.6700E-07
      | -2.8180E-05
      | -5.7027E-05
      | -8.5874E-05
      | -1.1472E-04],[9,4])
      settings: InputPortMap=u0,u1
  Z'uvw : Lookup_n-D  NumberOfTableDimensions=3  BreakpointsForDimension1=|  BreakpointsForDimension2=|  BreakpointsForDimension3=|  Table=|  InternalRulePriority=Speed  RndMeth=Simplest  InputSameDT=on
      BreakpointsForDimension1=|
      | [-24
      | -16
      | -8
      | 0
      | 8
      | 16
      | 24]
      BreakpointsForDimension2=|
      | [-5.1444E+00
      | -3.0866E+00
      | -1.5433E+00
      | ]
      Table=|
      | reshape([-7.6517E-03
      | -4.8509E-03
      | -2.1091E-03
      | 3.8840E-04
      | 2.9798E-03
      | 6.0809E-03
      | 8.2821E-03
      | -7.5270E-03
      | -4.7702E-03
      | -1.9652E-03
      | 3.8840E-04
      | 2.9512E-03
      | 6.0573E-03
      | 8.1333E-03
      | -7.5193E-03
      | -4.5800E-03
      | -1.6681E-03
      | 3.8840E-04
      | 2.7791E-03
      | 5.8231E-03
      | 8.3050E-03
      | -6.2244E-03
      | -3.6100E-03
      | -9.9571E-04
      | 1.6186E-03
      | 4.2329E-03
      | 6.8473E-03
      | 9.4616E-03
      | -5.2515E-03
      | -2.9614E-03
      | -6.7142E-04
      | 1.6186E-03
      | 3.9086E-03
      | 6.1987E-03
      | 8.4887E-03
      | -4.1283E-03
      | -2.2126E-03
      | -2.9701E-04
      | 1.6186E-03
      | 3.5342E-03
      | 5.4499E-03
      | 7.3655E-03
      | -6.1999E-03
      | -3.5260E-03
      | -8.5205E-04
      | 1.8219E-03
      | 4.4958E-03
      | 7.1698E-03
      | 9.8437E-03
      | -4.9811E-03
      | -2.7134E-03
      | -4.4577E-04
      | 1.8219E-03
      | 4.0896E-03
      | 6.3572E-03
      | 8.6249E-03
      | -5.2821E-03
      | -2.9141E-03
      | -5.4610E-04
      | 1.8219E-03
      | 4.1899E-03
      | 6.5579E-03
      | 8.9259E-03
      | -6.1195E-03
      | -3.4239E-03
      | -7.2823E-04
      | 1.9674E-03
      | 4.6630E-03
      | 7.3587E-03
      | 1.0054E-02
      | -4.7022E-03
      | -2.4512E-03
      | -2.0024E-04
      | 1.9674E-03
      | 4.2184E-03
      | 6.4693E-03
      | 8.7203E-03
      | -3.4515E-03
      | -1.6452E-03
      | 1.6111E-04
      | 1.9674E-03
      | 3.7737E-03
      | 5.5800E-03
      | 7.3863E-03],[7,3,4])
      BreakpointsForDimension3=|
      | [-35.0624 -18.3724 -15.3724 -13.8724
      | ]
      settings: InputPortMap=u0,u1,u2
  ZdXi : Subsystem
  Zqq : Lookup_n-D  NumberOfTableDimensions=1  BreakpointsForDimension1=|  Table=|  InternalRulePriority=Speed  RndMeth=Simplest  InputSameDT=on
      BreakpointsForDimension1=|
      | [-0.02
      | -0.015
      | -0.012958963
      | -0.009719222
      | -0.006479482
      | -0.003239741
      | -0.00161987
      | -0.000647948
      | 0.000647948
      | 0.00161987
      | 0.003239741
      | 0.006479482
      | 0.009719222
      | 0.012958963
      | 0.015
      | 0.02
      | ]
      Table=|
      | [3.6478E-03
      | 3.8686E-03
      | 3.4313E-03
      | 4.0790E-03
      | 3.9500E-03
      | 3.6018E-03
      | 3.6796E-03
      | 3.5502E-03
      | 3.4310E-03
      | 3.4872E-03
      | 4.2239E-03
      | 4.0934E-03
      | 3.0314E-03
      | 2.5726E-03
      | 2.9188E-03
      | 2.7740E-03
      | ]
  Zuq : Lookup_n-D  NumberOfTableDimensions=1  BreakpointsForDimension1=|  Table=|  InternalRulePriority=Speed  RndMeth=Simplest  InputSameDT=on
      BreakpointsForDimension1=|
      | [-0.04
      | -0.03
      | -0.02
      | -0.01
      | -0.005
      | -0.002
      | 0.002
      | 0.005
      | 0.01
      | 0.02
      | 0.03
      | 0.04
      | ]
      Table=|
      | [-9.8908E-03
      | -9.0784E-03
      | -8.9566E-03
      | -1.0733E-02
      | -1.4141E-02
      | -2.4189E-02
      | -6.5605E-03
      | -7.1594E-03
      | -7.6366E-03
      | -7.9008E-03
      | -6.1794E-03
      | -6.1029E-03
      | ]
  Zwq : Lookup_n-D  NumberOfTableDimensions=1  BreakpointsForDimension1=|  Table=|  InternalRulePriority=Speed  RndMeth=Simplest  InputSameDT=on
      BreakpointsForDimension1=|
      | [-0.0015
      | -0.0012
      | -0.0009
      | -0.0006
      | -0.0003
      | -0.0001
      | 0.0001
      | 0.0003
      | 0.0006
      | 0.0009
      | 0.0012
      | 0.0015]
      Table=|
      | [-2.9784E-01
      | -2.6725E-01
      | -2.3292E-01
      | -2.0077E-01
      | -1.1489E-01
      | -7.6673E-03
      | -7.5516E-03
      | -1.1617E-01
      | -2.0077E-01
      | -2.9128E-01
      | -3.5974E-01
      | -4.7839E-01]
  Z : Outport
  wires:
  Fz/3(FZstat) -> To Workspace2/1
  Fz/4(FZprop) -> To Workspace3/1
  Fz/5(FZhull) -> To Workspace4/1
  Fz/2(FZApp) -> To Workspace/1
  Z'uvw/1 -> Fz/7(Zuvw)
  Selector4/1 -> Z'uvw/3, ZdXi/2(z)
  Zvm/1 -> Fz/15(Zvm)
  Z'uq Prop/1 -> Fz/8(CZProp)
  Z'dwdt/1(Zdwdt) -> Fz/9(Zdwdt)
  ZdXi/1(ZdX) -> Fz/14(ZdXi)
  Zuq/1 -> Fz/5(Zuq)
  Zqq/1 -> Fz/4(Zqq)
  Fz/1(FZ) -> Z/1, To Workspace1/1
  Zwq/1 -> Fz/6(Zwq)
  Saturation3/1 -> Zqq/1
  Saturation2/1 -> Zwq/1
  Saturation1/1 -> Zuq/1
  dX/1 -> ZdXi/1(dX)
  Selector1/1 -> Z'dwdt/1(a3)
  dmass/1 -> Fz/13(dmass)
  dLCG/1 -> Fz/12(dLCG)
  Ba/1 -> Fz/3(Ba), Selector1/1
  Product1/1 -> Saturation2/1
  Selector3/1 -> Product1/2
  UeX/1 -> Fz/11(UeX)
  Product3/1 -> Z'uq Prop/1, Saturation1/1
  Bx/1 -> Fz/1(Bx), Selector4/1
  Umag/1 -> Fz/10(Umag)
  Bv/1 -> Fz/2(Bv), Selector2/1, Selector3/1, Selector7/1
  Alpha/1 -> Z'uvw/1
  Selector2/1 -> Product3/1, Saturation3/1, Product1/1
  Selector7/1 -> Product3/2, Z'uq Prop/2, Z'uvw/2

== system Model_6DOF_B3/HDM B3/Effective Veloicity Calclation ==
  Bv : Inport
  uwsXi : Inport  Port=2
  uwsCG : Inport  Port=3
  Add{,1..4} (5 alike) : Sum
  Demux : Demux  Outputs=5
  Demux1 : Demux  Outputs=3
  Demux2 : Demux  Outputs=5
  Gain : Gain
  Gain1 : Gain
  Gain2 : Gain
  MATLAB Function : MATLAB Function  TreatAsAtomicUnit=on
  MATLAB Function1 : MATLAB Function  TreatAsAtomicUnit=on
  MATLAB Function2 : MATLAB Function  TreatAsAtomicUnit=on
  X_SP1 : Constant  Value=[31.924; 3.861; -3.861;]
  X_SP2 : Constant  Value=[31.924; 3.861; 3.861;]
  X_SP3 : Constant  Value=[31.924; -3.861; 3.861;]
  X_SP4 : Constant  Value=[31.924; -3.861; -3.861;]
  X_XB : Constant  Value=[-10.465; 0; 9.732;]
  aX : Scope  NumInputPorts=5
  n1 : Constant  Value=[0; 1/sqrt(2); -1/sqrt(2);]
  n2 : Constant  Value=[0; 1/sqrt(2); 1/sqrt(2);]
  n3 : Constant  Value=[0; -1/sqrt(2); 1/sqrt(2);]
  n4 : Constant  Value=[0; -1/sqrt(2); -1/sqrt(2);]
  n5 : Constant  Value=[0; 1; 0;]
  nh : Constant  Value=[-1; 0; 0;]
  urXi : Scope  NumInputPorts=5
  Alpha : Outport
  Beta : Outport  Port=2
  Umag : Outport  Port=3
  aXi : Outport  Port=4
  UeX : Outport  Port=5
  wires:
  Bv/1 -> MATLAB Function1/6(U_ship), MATLAB Function2/1(Bv)
  nh/1 -> MATLAB Function/1(nh)
  n1/1 -> MATLAB Function/2(n1)
  n2/1 -> MATLAB Function/3(n2)
  n3/1 -> MATLAB Function/4(n3)
  n4/1 -> MATLAB Function/5(n4)
  X_XB/1 -> MATLAB Function1/5(rXB)
  X_SP2/1 -> MATLAB Function1/2(rX2)
  X_SP3/1 -> MATLAB Function1/3(rX3)
  X_SP4/1 -> MATLAB Function1/4(rX4)
  X_SP1/1 -> MATLAB Function1/1(rX1)
  n5/1 -> MATLAB Function/6(nB)
  MATLAB Function1/1(urX1) -> Add/1, urXi/1
  MATLAB Function/1(aX) -> Gain1/1, Demux2/1
  Demux/1 -> Add/2
  Add/1 -> MATLAB Function/7(urX1)
  Add1/1 -> MATLAB Function/8(urX2)
  Add2/1 -> MATLAB Function/9(urX3)
  Add3/1 -> MATLAB Function/10(urX4)
  Add4/1 -> MATLAB Function/11(urXB)
  Demux/2 -> Add1/2
  Demux/3 -> Add2/2
  Demux/4 -> Add3/2
  Demux/5 -> Add4/2
  MATLAB Function1/5(urXB) -> Add4/1, urXi/5
  MATLAB Function1/4(urX4) -> Add3/1, urXi/4
  MATLAB Function1/3(urX3) -> Add2/1, urXi/3
  MATLAB Function1/2(urX2) -> Add1/1, urXi/2
  MATLAB Function2/1(alpha) -> Gain/1
  MATLAB Function2/2(beta) -> Beta/1
  MATLAB Function2/3(Umag) -> Umag/1
  MATLAB Function/2(UeX) -> UeX/1
  Demux1/1 -> MATLAB Function2/2(uCG)
  Demux1/2 -> MATLAB Function2/3(vCG)
  Demux1/3 -> MATLAB Function2/4(wCG)
  Demux2/1 -> aX/1
  Demux2/2 -> aX/2
  Demux2/3 -> aX/3
  Demux2/4 -> aX/4
  Demux2/5 -> aX/5
  uwsCG/1 -> Demux1/1
  Gain/1 -> Alpha/1
  Gain1/1 -> aXi/1
  Gain2/1 -> Demux/1
  uwsXi/1 -> Gain2/1

== system Model_6DOF_B3/HDM B3/Effective dX Calculation ==
  dX CTRL : Inport
  aXi : Inport  Port=2
  Add{,1..4} (5 alike) : Sum
  Demux : Demux  Outputs=5
  Demux1 : Demux  Outputs=5
  Mux6 : Mux  Inputs=5
  dXeff : Outport
  wires:
  dX CTRL/1 -> Demux/1
  aXi/1 -> Demux1/1
  Add/1 -> Mux6/1
  Add1/1 -> Mux6/2
  Add2/1 -> Mux6/3
  Add3/1 -> Mux6/4
  Add4/1 -> Mux6/5
  Demux/1 -> Add/1
  Demux/2 -> Add1/1
  Demux/3 -> Add2/1
  Demux/4 -> Add3/1
  Demux/5 -> Add4/1
  Demux1/1 -> Add/2
  Demux1/2 -> Add1/2
  Demux1/3 -> Add2/2
  Demux1/4 -> Add3/2
  Demux1/5 -> Add4/2
  Mux6/1 -> dXeff/1

== system Model_6DOF_B3/HDM B3/K ==
  Bx : Inport
  Bv : Inport  Port=2
  Ba : Inport  Port=3
  Beta : Inport  Port=4
  Umag : Inport  Port=5
  dX : Inport  Port=6
  UeX : Inport  Port=7
  dLCG : Inport  Port=8
  dmass : Inport  Port=9
  Kvm : Inport  Port=10
  BFM : Inport  Port=11
  Abs : Abs
  Abs1 : Abs
  Abs2 : Abs
  Gain : Gain
  Gain1 : Gain
  Gain2 : Gain
  Gain3 : Gain  Gain=-1
  K'p|p| : Lookup_n-D  NumberOfTableDimensions=1  BreakpointsForDimension1=|  Table=|  InternalRulePriority=Speed  RndMeth=Simplest  InputSameDT=on
      BreakpointsForDimension1=|
      | [-0.0015
      | -0.0012
      | -0.0009
      | -0.0006
      | -0.0003
      | -0.0001
      | 0.0001
      | 0.0003
      | 0.0006
      | 0.0009
      | 0.0012
      | 0.0015]
      Table=|
      | [-1.3011E-02
      | -1.6962E-02
      | -2.0682E-02
      | -3.1419E-02
      | -6.4407E-02
      | -1.9322E-01
      | 1.9322E-01
      | 6.4378E-02
      | 3.1944E-02
      | 2.1072E-02
      | 1.6415E-02
      | 1.3407E-02]
  K'up : Lookup_n-D  NumberOfTableDimensions=1  BreakpointsForDimension1=|  Table=|  InternalRulePriority=Speed  RndMeth=Simplest  InputSameDT=on
      BreakpointsForDimension1=|
      | [0.03999989
      | 0.079999993
      | 0.11999963
      | 0.15999956]
      Table=|
      | [-4.0344E-04
      | -8.1402E-04
      | -1.2116E-03
      | -1.6125E-03]
  K'ur : Lookup_n-D  NumberOfTableDimensions=1  BreakpointsForDimension1=|  Table=|  InternalRulePriority=Speed  RndMeth=Simplest  InputSameDT=on
      BreakpointsForDimension1=|
      | [-0.0015
      | -0.0012
      | -0.0009
      | -0.0006
      | -0.0003
      | -0.0001
      | 0.0001
      | 0.0003
      | 0.0006
      | 0.0009
      | 0.0012
      | 0.0015]
      Table=|
      | [-1.3011E-02
      | -1.6962E-02
      | -2.0682E-02
      | -3.1419E-02
      | -6.4407E-02
      | -1.9322E-01
      | 1.9322E-01
      | 6.4378E-02
      | 3.1944E-02
      | 2.1072E-02
      | 1.6415E-02
      | 1.3407E-02]
  K'uvw : Lookup_n-D  NumberOfTableDimensions=3  BreakpointsForDimension1=|  BreakpointsForDimension2=|  BreakpointsForDimension3=|  Table=|  InternalRulePriority=Speed  RndMeth=Simplest  InputSameDT=on
      BreakpointsForDimension1=|
      | [0
      | 4
      | 8
      | 12]
      BreakpointsForDimension2=|
      | [-5.1444E+00
      | -3.0866E+00
      | -1.5433E+00
      | ]
      Table=|
      | reshape([0.0000000E+00
      | 1.5570290E-04
      | 3.7677829E-04
      | 6.0025374E-04
      | 0.0000000E+00
      | 1.5575678E-04
      | 3.8557685E-04
      | 6.0103850E-04
      | 0.0000000E+00
      | 1.7511088E-04
      | 3.8376789E-04
      | 6.0108480E-04
      | 0.0000000E+00
      | 1.9071552E-04
      | 4.0986649E-04
      | 6.4012030E-04
      | 0.0000000E+00
      | 1.8940622E-04
      | 4.0946931E-04
      | 6.3613461E-04
      | 0.0000000E+00
      | 1.8621071E-04
      | 4.0619654E-04
      | 7.0286379E-04
      | 0.0000000E+00
      | 2.0712189E-04
      | 4.4751988E-04
      | 7.0514631E-04
      | 0.0000000E+00
      | 1.9895751E-04
      | 4.3099356E-04
      | 6.6994571E-04
      | 0.0000000E+00
      | 1.9568554E-04
      | 4.2679977E-04
      | 6.6445067E-04
      | 0.0000000E+00
      | 2.4359563E-04
      | 5.3740096E-04
      | 8.5879902E-04
      | 0.0000000E+00
      | 2.0890025E-04
      | 4.5502130E-04
      | 7.1388224E-04
      | 0.0000000E+00
      | 2.0575072E-04
      | 4.5505766E-04
      | 7.0285206E-04],[4,3,4])
      BreakpointsForDimension3=|
      | [-35.0624 -18.3724 -15.3724 -13.8724
      | ]
      settings: InputPortMap=u0,u1,u2
  KdXi : Subsystem
  Mux : Mux  Inputs=7
  Mx : MATLAB Function  TreatAsAtomicUnit=on
  Product{,1..2,4..5} (5 alike) : Product
  Saturation4 : Saturate  UpperLimit=-13.8724  LowerLimit=-35.0624
  Scope : Scope
  Selector1 : Selector  InputPortWidth=6  IndexOptions=Index vector (dialog)  Indices=4  OutputSizes=1
  Selector10 : Selector  InputPortWidth=6  IndexOptions=Index vector (dialog)  Indices=1  OutputSizes=1
  Selector2 : Selector  InputPortWidth=6  IndexOptions=Index vector (dialog)  Indices=3  OutputSizes=1
  Selector4 : Selector  InputPortWidth=6  IndexOptions=Index vector (dialog)  Indices=4  OutputSizes=1
  Selector8 : Selector  InputPortWidth=6  IndexOptions=Index vector (dialog)  Indices=2  OutputSizes=1
  Sign : Signum
  Sign1 : Signum
  To Workspace : ToWorkspace  VariableName=K_total  SaveFormat=Timeseries  SampleTime=-1
  To Workspace1 : ToWorkspace  VariableName=AppK_All  SaveFormat=Timeseries  SampleTime=-1
  To Workspace2 : ToWorkspace  VariableName=KHullVM  SaveFormat=Timeseries  SampleTime=-1
  To Workspace3 : ToWorkspace  VariableName=Kvm  SaveFormat=Timeseries  SampleTime=-1
  To Workspace8 : ToWorkspace  VariableName=Benchmark_K  SaveFormat=Timeseries  SampleTime=-1
  K : Outport
  wires:
  Bv/1 -> Selector10/1, Selector4/1, Selector8/1, Mx/2(Bv)
  Bx/1 -> Mx/1(Bx), Selector2/1
  Selector10/1 -> K'uvw/2, Product1/1
  Ba/1 -> Mx/3(Ba)
  UeX/1 -> KdXi/2(UeX), Mx/9(UeX)
  Beta/1 -> Sign1/1, Abs2/1
  Umag/1 -> Mx/8(Umag)
  dLCG/1 -> Mx/10(dLCG)
  dmass/1 -> Mx/11(dmass)
  dX/1 -> KdXi/1(dX)
  K'up/1 -> Product/2
  K'p|p|/1 -> Gain2/1
  Product4/1 -> K'ur/1
  Selector8/1 -> Product4/1
  Abs/1 -> Product5/1
  Product5/1 -> K'p|p|/1
  Selector4/1 -> Product1/2, Product5/2, Abs/1, Product4/2
  K'ur/1 -> Mx/6(CKpp)
  KdXi/1(KdXi) -> Mx/12(CNdXi)
  Selector2/1 -> Saturation4/1
  K'uvw/1 -> Product2/2
  Product1/1 -> Sign/1, Abs1/1
  Abs1/1 -> K'up/1
  Sign/1 -> Product/1
  Product/1 -> Gain1/1
  Product2/1 -> Mx/7(CKuvw)
  Abs2/1 -> K'uvw/1
  Sign1/1 -> Gain/1
  Mux/1 -> To Workspace8/1
  Mx/2(KApp) -> Mux/1
  Mx/3(K_hull) -> Mux/2
  Mx/4(Kh_total) -> Mux/3
  Mx/5(Kpp) -> Mux/4
  Mx/6(KAppAll) -> To Workspace1/1
  BFM/1 -> Selector1/1
  Selector1/1 -> Mx/14(BFK)
  Mx/1(K) -> Scope/1, Mux/6, To Workspace/1, K/1
  Mx/7(KStat) -> [K_Stat]
  Gain/1 -> Product2/1
  Gain1/1 -> Mx/4(CKup)
  Gain2/1 -> Mx/5(CKur)
  [K_Stat] -> Mux/7
  Saturation4/1 -> KdXi/3(z), K'uvw/3  "z"
  Mx/8(KHullVM) -> To Workspace2/1
  Kvm/1 -> Gain3/1
  Gain3/1 -> Mx/13(Kvm), To Workspace3/1, Mux/5
